simulink model "attempt_2_Full_Microthruster_Simulation"  (R2021b)
settings: Solver=ode45  StartTime=0.0  StopTime=simtime  RelTol=1e-16  AbsTol=1e-16
undefined symbols (not defined in the file): delta_t, dev_en, drag_unmodeled, dtype_g, euler_b_ECI0, euler_b_LVLH0, euler_LVLH_ECI0, g_bias, g_sath, g_satl, g_sen, g_sf_cc, geom, gr_eff_unmodeled, grav_grad_unmodeled, gyro_meas_frequ, J, JD_start, mag_field_unmodeled, mag_meas_frequ, mu, onboard_unmodeled, quat_b_ECI0, quat_b_LVLH0, quat_LVLH_ECI0, r, sigma_g, sigma_m, sigma_q, sigma_s, srp_unmodeled, sun_meas_frequ, theor_torque, ts, v, w_b_ECI0, wn, zn
libraries: aerolibnav x5, sharedTrackingLibrary x2
(part 1 of 2)
settings Model: Creator=Owner  LastModifiedBy=Owner
settings DebuggingCC: UnderSpecifiedDimensionMsg=warning

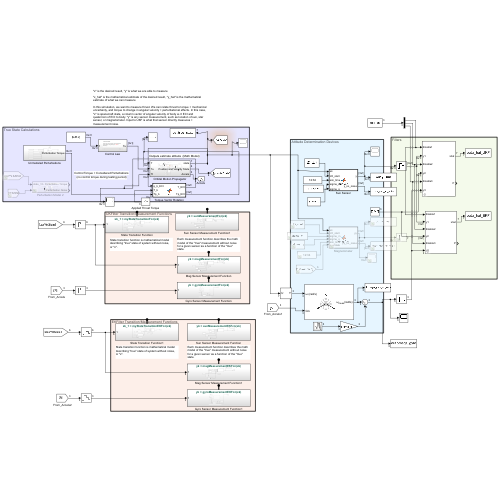
[thumbnail: Simulink's stored preview of the top-level diagram]
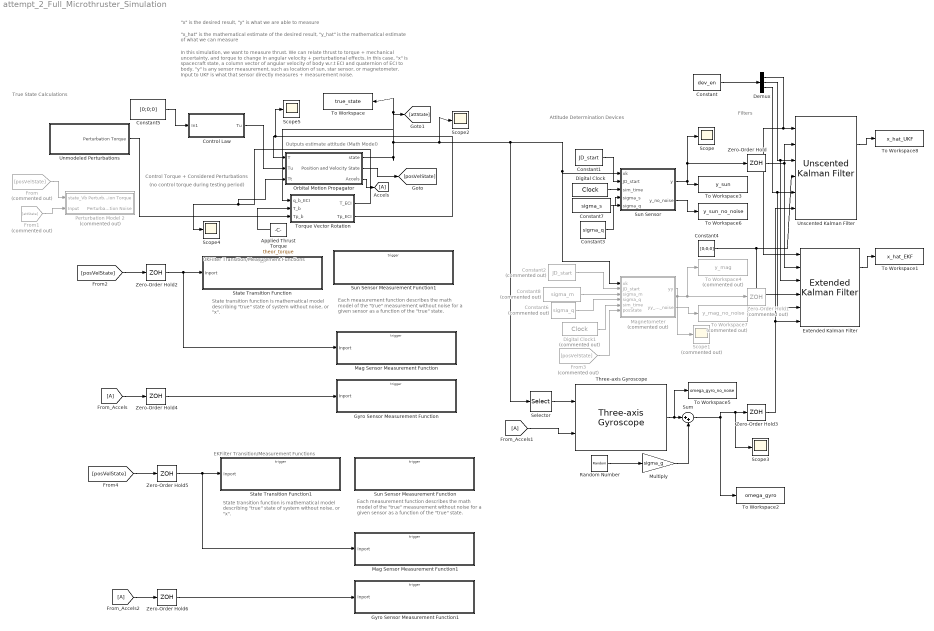
== system attempt_2_Full_Microthruster_Simulation ==
  note: Filters
  note: Attitude Determination Devices
  note: UKFilter Transition/Measurement Functions
  note: True State Calculations
  note: Each measurement function describes the math model of the "true" measurement without noise for a given sensor as a function of the "true" state.
  note: State transition function is mathematical model describing "true" state of system without noise, or "x".
  note: In this simulation, we want to measure thrust. We can relate thrust to torque + mechanical uncertainty, and torque to change in angular velocity + perturbational effects. In this case, "x" is spacecraft state, a column vector of angular velocity of body w.r.t ECI and quaternion of ECI to body. "y" is any sensor measurement, such as location of sun, star sensor, or magnetometer. Input to UKF is what that sensor directly measures + measurement noise.
  note: "x_hat" is the mathematical estimate of the desired result, "y_hat" is the mathematical estimate of what we can measure
  note: "x" is the desired result, "y" is what we are able to measure
  note: Outputs estimate attitude (Math Model)
  note: (no control torque during testing period)
  note: Control Torque + Considered Perturbations
  note: State transition function is mathematical model describing "true" state of system without noise, or "x".
  note: Each measurement function describes the math model of the "true" measurement without noise for a given sensor as a function of the "true" state.
  note: EKFilter Transition/Measurement Functions
  Applied Thrust Torque : Constant  Value=theor_torque
  Constant : Constant  Value=dev_en
  Constant1 : Constant  Value=JD_start
  Constant2 : Constant  Commented=on  Value=JD_start
  Constant3 : Constant  Value=sigma_q
  Constant4 : Constant  Value=[0;0;0]
  Constant5 : Constant  Value=[0;0;0]  VectorParams1D=off
  Constant6 : Constant  Commented=on  Value=sigma_q
  Constant7 : Constant  Value=sigma_s  VectorParams1D=off
  Constant8 : Constant  Commented=on  Value=sigma_m  VectorParams1D=off
  Control Law : Subsystem
  Demux : Demux  Outputs=3
  Digital Clock : DigitalClock  SampleTime=delta_t
  Digital Clock1 : DigitalClock  Commented=on  SampleTime=delta_t
  Extended Kalman Filter : sharedTrackingLibrary/Extended Kalman Filter  StateTransitionFcn=myStateTransitionEKFcn  HasStateTransitionJacobianFcn=off  HasAdditiveProcessNoise=Additive  ProcessNoise=Q_k  HasTimeVaryingProcessNoise=off  HasStateTransitionFcnExtraArgument=0  InitialState=x_hat0  InitialStateCovariance=P0  MeasurementFcn1=sunMeasurementEKFcn  HasMeasurementJacobianFcn1=off  HasMeasurementEnablePort1=on  HasAdditiveMeasurementNoise1=Additive  MeasurementNoise1=R_k  HasTimeVaryingMeasurementNoise1=off  HasMeasurementFcnExtraArgument1=0  MeasurementFcn2=magMeasurementEKFcn  HasMeasurementJacobianFcn2=off  HasMeasurementEnablePort2=on  HasAdditiveMeasurementNoise2=Additive  MeasurementNoise2=RR_k  HasTimeVaryingMeasurementNoise2=off  HasMeasurementFcnExtraArgument2=0  MeasurementFcn3=gyroMeasurementEKFcn  HasMeasurementJacobianFcn3=off  HasMeasurementEnablePort3=on  HasAdditiveMeasurementNoise3=Additive  MeasurementNoise3=RRR_k  HasTimeVaryingMeasurementNoise3=off  HasMeasurementFcnExtraArgument3=0  MeasurementFcn4=myMeasurementFcn  HasMeasurementJacobianFcn4=off  HasMeasurementEnablePort4=off  HasAdditiveMeasurementNoise4=Additive  MeasurementNoise4=1  HasTimeVaryingMeasurementNoise4=off  HasMeasurementFcnExtraArgument4=0  MeasurementFcn5=myMeasurementFcn  HasMeasurementJacobianFcn5=off  HasMeasurementEnablePort5=off  HasAdditiveMeasurementNoise5=Additive  MeasurementNoise5=1  HasTimeVaryingMeasurementNoise5=off  HasMeasurementFcnExtraArgument5=0  EnableMultirate=on  StateTransitionFcnSampleTime=delta_t  MeasurementFcn1SampleTime=1/sun_meas_frequ  MeasurementFcn2SampleTime=1/mag_meas_frequ  MeasurementFcn3SampleTime=1/gyro_meas_frequ  MeasurementFcn4SampleTime=1  MeasurementFcn5SampleTime=1  UseCurrentEstimator=on  OutputStateCovariance=on  DataType=double  SampleTime=delta_t  NumberOfMeasurements=3
      settings: SourceProductBaseCode=AE,PW,CT,DR,TF,ID,LP,NV,AR,RO,RR,UV,VE
  From : From  Commented=on  GotoTag=posVelState
  From1 : From  Commented=on  GotoTag=attState
  From3 : From  Commented=on  GotoTag=posVelState
  Gyro Sensor Measurement Function : Subsystem  TreatAsAtomicUnit=on
  Gyro Sensor Measurement Function1 : Subsystem  TreatAsAtomicUnit=on
  Mag Sensor Measurement Function : Subsystem  TreatAsAtomicUnit=on
  Mag Sensor Measurement Function1 : Subsystem  TreatAsAtomicUnit=on
  Magnetometer : MATLAB Function  Commented=on  TreatAsAtomicUnit=on
  Multiply : Gain  Gain=sigma_g
  Orbital Motion Propagator : Subsystem
  Perturbation Model 2 : Subsystem  Commented=on
  Random Number : RandomNumber  Seed=[0 0 0]
  Scope{,2..5} (5 alike) : Scope
  Scope1 : Scope  Commented=on
  Selector : Selector  InputPortWidth=7  IndexOptions=Index vector (dialog)  Indices=[1 2 3]  OutputSizes=1
  State Transition Function : Subsystem  TreatAsAtomicUnit=on
  State Transition Function1 : Subsystem  TreatAsAtomicUnit=on
  Sum : Sum  Inputs=|++
  Sun Sensor : MATLAB Function  TreatAsAtomicUnit=on
  Sun Sensor Measurement Function : Subsystem  TreatAsAtomicUnit=on
  Sun Sensor Measurement Function1 : Subsystem  TreatAsAtomicUnit=on
  Three-axis Gyroscope : aerolibnav/Three-axis Gyroscope  dtype_g=off  w_g=190  z_g=0.707  g_sf_cc=[1 0 0; 0 1 0; 0 0 1]  g_bias=[0 0 0]  g_sen=[0 0 0]  g_Ts=0  g_rand=off  g_seeds=[23093 23094 23095]  g_pow=[sigma_g sigma_g sigma_g]  g_sat="[-inf  -inf  -inf  inf inf inf]"
      settings: SourceProductBaseCode=AE
  To Workspace : ToWorkspace  VariableName=true_state  SaveFormat=Timeseries  SampleTime=-1
  To Workspace1 : ToWorkspace  VariableName=x_hat_EKF  SaveFormat=Timeseries  SampleTime=-1
  To Workspace2 : ToWorkspace  VariableName=omega_gyro  SaveFormat=Timeseries  SampleTime=-1
  To Workspace3 : ToWorkspace  VariableName=y_sun  SaveFormat=Timeseries  SampleTime=-1
  To Workspace4 : ToWorkspace  Commented=on  VariableName=y_mag  SaveFormat=Timeseries  SampleTime=-1
  To Workspace5 : ToWorkspace  VariableName=omega_gyro_no_noise  SaveFormat=Timeseries  SampleTime=-1
  To Workspace6 : ToWorkspace  VariableName=y_sun_no_noise  SaveFormat=Timeseries  SampleTime=-1
  To Workspace7 : ToWorkspace  Commented=on  VariableName=y_mag_no_noise  SaveFormat=Timeseries  SampleTime=-1
  To Workspace8 : ToWorkspace  VariableName=x_hat_UKF  SaveFormat=Timeseries  SampleTime=-1
  Torque Vector Rotation : MATLAB Function  TreatAsAtomicUnit=on
  Unmodeled Perturbations : Subsystem
  Unscented Kalman Filter : sharedTrackingLibrary/Unscented Kalman Filter  StateTransitionFcn=myStateTransitionFcn  HasAdditiveProcessNoise=Additive  ProcessNoise=Q_k  HasTimeVaryingProcessNoise=off  HasStateTransitionFcnExtraArgument=0  InitialState=x_hat0  InitialStateCovariance=P0  Alpha=1e-5  Beta=2  Kappa=0  MeasurementFcn1=sunMeasurementFcn  HasMeasurementEnablePort1=on  HasAdditiveMeasurementNoise1=Additive  MeasurementNoise1=R_k  HasTimeVaryingMeasurementNoise1=off  HasMeasurementFcnExtraArgument1=0  MeasurementFcn2=magMeasurementFcn  HasMeasurementEnablePort2=on  HasAdditiveMeasurementNoise2=Additive  MeasurementNoise2=RR_k  HasTimeVaryingMeasurementNoise2=off  HasMeasurementFcnExtraArgument2=0  MeasurementFcn3=gyroMeasurementFcn  HasMeasurementEnablePort3=on  HasAdditiveMeasurementNoise3=Additive  MeasurementNoise3=RRR_k  HasTimeVaryingMeasurementNoise3=off  HasMeasurementFcnExtraArgument3=0  MeasurementFcn4=myMeasurementFcn  HasMeasurementEnablePort4=off  HasAdditiveMeasurementNoise4=Nonadditive  MeasurementNoise4=1  HasTimeVaryingMeasurementNoise4=off  HasMeasurementFcnExtraArgument4=0  MeasurementFcn5=myMeasurementFcn  HasMeasurementEnablePort5=off  HasAdditiveMeasurementNoise5=Additive  MeasurementNoise5=1  HasTimeVaryingMeasurementNoise5=off  HasMeasurementFcnExtraArgument5=0  EnableMultirate=on  StateTransitionFcnSampleTime=delta_t  MeasurementFcn1SampleTime=1/sun_meas_frequ  MeasurementFcn2SampleTime=1/mag_meas_frequ  MeasurementFcn3SampleTime=1/gyro_meas_frequ  MeasurementFcn4SampleTime=1  MeasurementFcn5SampleTime=1  UseCurrentEstimator=on  OutputStateCovariance=on  DataType=double  SampleTime=delta_t  NumberOfMeasurements=3
      settings: SourceProductBaseCode=AE,PW,CT,DR,TF,ID,LP,NV,AR,RO,RR,UV,VE
  Zero-Order Hold : ZeroOrderHold  SampleTime=1/sun_meas_frequ
  Zero-Order Hold1 : ZeroOrderHold  Commented=on  SampleTime=1/mag_meas_frequ
  Zero-Order Hold{2,4..6} (4 alike) : ZeroOrderHold  SampleTime=-1
  Zero-Order Hold3 : ZeroOrderHold  SampleTime=1/gyro_meas_frequ
  wires:
  Control Law/1(Tu) -> Orbital Motion Propagator/2(Tu)
  Constant/1 -> Demux/1
  Applied Thrust Torque/1 -> Torque Vector Rotation/2(T_b)
  Torque Vector Rotation/1(T_ECI) -> Orbital Motion Propagator/3(Tt), Scope4/1
  Orbital Motion Propagator/1(state) -> Torque Vector Rotation/1(q_b_ECI), Scope2/1, Selector/1, Sun Sensor/1(xk), Magnetometer/1(xk), [attState], To Workspace/1
  Zero-Order Hold/1 -> Extended Kalman Filter/2, Unscented Kalman Filter/2
  Digital Clock/1 -> Sun Sensor/3(sim_time)
  Constant7/1 -> Sun Sensor/4(sigma_s)
  Constant1/1 -> Sun Sensor/2(JD_start)
  Constant3/1 -> Sun Sensor/5(sigma_q)
  Sun Sensor/1(y) -> To Workspace3/1, Scope/1, Zero-Order Hold/1
  Unscented Kalman Filter/1 -> To Workspace8/1
  Extended Kalman Filter/1 -> To Workspace1/1
  Constant6/1 -> Magnetometer/4(sigma_q)
  Constant8/1 -> Magnetometer/3(sigma_m)
  Magnetometer/1(yy) -> Scope1/1, Zero-Order Hold1/1, To Workspace4/1
  Orbital Motion Propagator/2(Position and Velocity State) -> [posVelState]
  From/1 -> Perturbation Model 2/1(state_Vb)
  From1/1 -> Perturbation Model 2/2(Input)
  [posVelState] -> Zero-Order Hold2/1
  Digital Clock1/1 -> Magnetometer/5(sim_time)
  From3/1 -> Magnetometer/6(posState)
  Zero-Order Hold2/1 -> Mag Sensor Measurement Function/1(Inport), State Transition Function/1(Inport)
  Constant5/1 -> Control Law/1(In1)
  Selector/1 -> Three-axis Gyroscope/1
  Zero-Order Hold3/1 -> Unscented Kalman Filter/6, Extended Kalman Filter/6
  Orbital Motion Propagator/3(Accels) -> [A]
  [A] -> Zero-Order Hold4/1
  Zero-Order Hold4/1 -> Gyro Sensor Measurement Function/1(Inport)
  [A] -> Three-axis Gyroscope/2
  Zero-Order Hold6/1 -> Gyro Sensor Measurement Function1/1(Inport)
  Zero-Order Hold5/1 -> Mag Sensor Measurement Function1/1(Inport), State Transition Function1/1(Inport)
  [A] -> Zero-Order Hold6/1
  [posVelState] -> Zero-Order Hold5/1
  Random Number/1 -> Multiply/1
  Multiply/1 -> Sum/2
  Three-axis Gyroscope/1 -> To Workspace5/1, Sum/1
  Sum/1 -> Scope3/1, Zero-Order Hold3/1, To Workspace2/1
  Constant2/1 -> Magnetometer/2(JD_start)
  Sun Sensor/2(y_no_noise) -> To Workspace6/1
  Magnetometer/2(yy_no_noise) -> To Workspace7/1
  Demux/3 -> Unscented Kalman Filter/5, Extended Kalman Filter/5
  Demux/2 -> Extended Kalman Filter/3, Unscented Kalman Filter/3
  Demux/1 -> Unscented Kalman Filter/1, Extended Kalman Filter/1
  Unmodeled Perturbations/1(Perturbation Torque) -> Torque Vector Rotation/3(Tp_b)
  Torque Vector Rotation/2(Tp_ECI) -> Scope5/1, Orbital Motion Propagator/1(T)
  Constant4/1 -> Unscented Kalman Filter/4, Extended Kalman Filter/4

== system attempt_2_Full_Microthruster_Simulation/Control Law ==
  note: PLACEHOLDER:
      |
      | Likely only control device on board will be impermanent magnetorquer; TBM if necessary
  In1 : Inport
  Tu : Outport
  wires:
  In1/1 -> Tu/1

== system attempt_2_Full_Microthruster_Simulation/Gyro Sensor Measurement Function ==
  note: Identical to "three-axis gyroscope" block, except modified to inherit sample time
  Inport : Inport
  gyroMeasurementFcn : TriggerPort  TriggerType=function-call  IsSimulinkFunction=on  FunctionName=gyroMeasurementFcn  FunctionVisibility=scoped  VariantControl=(inherit)
  Scope : Scope
  Selector : Selector  InputPortWidth=7  IndexOptions=Index vector (dialog)  Indices=[1 2 3]  OutputSizes=1
  Subsystem : Subsystem
  Three-axis Gyroscope : aerolibnav/Three-axis Gyroscope  Commented=on  dtype_g=on  w_g=190  z_g=0.707  g_sf_cc=[1 0 0; 0 1 0; 0 0 1]  g_bias=[0 0 0]  g_sen=[0 0 0]  g_Ts=1/gyro_meas_frequ  g_rand=off  g_seeds=[23093 23094 23095]  g_pow=[0.0001 0.0001 0.0001]  g_sat="[-inf  -inf  -inf  inf inf inf]"
      settings: SourceProductBaseCode=AE
  To Workspace : ToWorkspace  VariableName=y_UKF_gyro  SaveFormat=Timeseries  SampleTime=-1
  xk : ArgIn  DisableCoverage=on  PortDimensions=[7 1]  ArgumentName=xk
  yk : ArgOut  DisableCoverage=on  PortDimensions=[3 1]  ArgumentName=yk
  wires:
  Selector/1 -> Subsystem/1(p q r)
  xk/1 -> Selector/1
  Inport/1 -> Subsystem/2(G's)
  Subsystem/1((p q r)_meas) -> Scope/1, To Workspace/1, yk/1

== system attempt_2_Full_Microthruster_Simulation/Gyro Sensor Measurement Function1 ==
  note: Identical to "three-axis gyroscope" block, except modified to inherit sample time
  Inport : Inport
  gyroMeasurementEKFcn : TriggerPort  TriggerType=function-call  IsSimulinkFunction=on  FunctionName=gyroMeasurementEKFcn  FunctionVisibility=scoped  VariantControl=(inherit)
  Scope : Scope
  Selector : Selector  InputPortWidth=7  IndexOptions=Index vector (dialog)  Indices=[1 2 3]  OutputSizes=1
  Subsystem : Subsystem
  Three-axis Gyroscope : aerolibnav/Three-axis Gyroscope  Commented=on  dtype_g=on  w_g=190  z_g=0.707  g_sf_cc=[1 0 0; 0 1 0; 0 0 1]  g_bias=[0 0 0]  g_sen=[0 0 0]  g_Ts=1/gyro_meas_frequ  g_rand=off  g_seeds=[23093 23094 23095]  g_pow=[0.0001 0.0001 0.0001]  g_sat="[-inf  -inf  -inf  inf inf inf]"
      settings: SourceProductBaseCode=AE
  To Workspace : ToWorkspace  VariableName=y_EKF_gyro  SaveFormat=Timeseries  SampleTime=-1
  xk : ArgIn  DisableCoverage=on  PortDimensions=[7 1]  ArgumentName=xk
  yk : ArgOut  DisableCoverage=on  PortDimensions=[3 1]  ArgumentName=yk
  wires:
  Selector/1 -> Subsystem/1(p q r)
  xk/1 -> Selector/1
  Inport/1 -> Subsystem/2(G's)
  Subsystem/1((p q r)_meas) -> Scope/1, To Workspace/1, yk/1

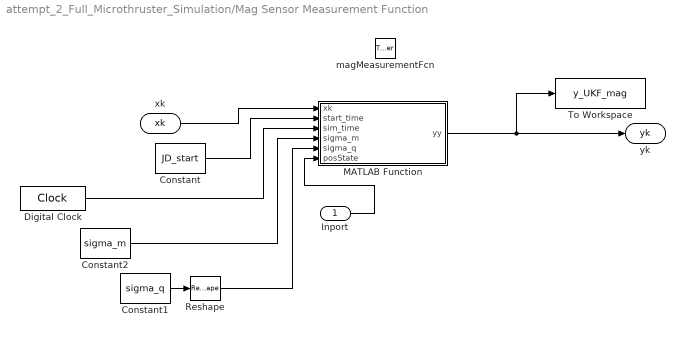
== system attempt_2_Full_Microthruster_Simulation/Mag Sensor Measurement Function ==
  Inport : Inport
  magMeasurementFcn : TriggerPort  TriggerType=function-call  IsSimulinkFunction=on  FunctionName=magMeasurementFcn  FunctionVisibility=scoped  VariantControl=(inherit)
  Constant : Constant  Value=JD_start
  Constant1 : Constant  Value=sigma_q  VectorParams1D=off  SampleTime=-1
  Constant2 : Constant  Value=sigma_m  VectorParams1D=off  SampleTime=-1
  Digital Clock : DigitalClock  SampleTime=-1
  MATLAB Function : MATLAB Function  TreatAsAtomicUnit=on
  Reshape : Reshape
  To Workspace : ToWorkspace  VariableName=y_UKF_mag  SaveFormat=Timeseries  SampleTime=-1
  xk : ArgIn  DisableCoverage=on  PortDimensions=[7 1]  ArgumentName=xk
  yk : ArgOut  DisableCoverage=on  PortDimensions=[3 1]  ArgumentName=yk
  wires:
  xk/1 -> MATLAB Function/1(xk)
  MATLAB Function/1(yy) -> To Workspace/1, yk/1
  Constant/1 -> MATLAB Function/2(start_time)
  Digital Clock/1 -> MATLAB Function/3(sim_time)
  Constant2/1 -> MATLAB Function/4(sigma_m)
  Constant1/1 -> Reshape/1
  Reshape/1 -> MATLAB Function/5(sigma_q)
  Inport/1 -> MATLAB Function/6(posState)

== system attempt_2_Full_Microthruster_Simulation/Mag Sensor Measurement Function1 ==
  Inport : Inport
  magMeasurementEKFcn : TriggerPort  TriggerType=function-call  IsSimulinkFunction=on  FunctionName=magMeasurementEKFcn  FunctionVisibility=scoped  VariantControl=(inherit)
  Constant : Constant  Value=JD_start
  Constant1 : Constant  Value=sigma_q  VectorParams1D=off  SampleTime=-1
  Constant2 : Constant  Value=sigma_m  VectorParams1D=off  SampleTime=-1
  Digital Clock : DigitalClock  SampleTime=-1
  MATLAB Function : MATLAB Function  TreatAsAtomicUnit=on
  Reshape : Reshape
  To Workspace : ToWorkspace  VariableName=y_EKF_mag  SaveFormat=Timeseries  SampleTime=-1
  xk : ArgIn  DisableCoverage=on  PortDimensions=[7 1]  ArgumentName=xk
  yk : ArgOut  DisableCoverage=on  PortDimensions=[3 1]  ArgumentName=yk
  wires:
  xk/1 -> MATLAB Function/1(xk)
  MATLAB Function/1(yy) -> To Workspace/1, yk/1
  Constant/1 -> MATLAB Function/2(JD_start)
  Digital Clock/1 -> MATLAB Function/3(sim_time)
  Constant2/1 -> MATLAB Function/4(sigma_m)
  Constant1/1 -> Reshape/1
  Reshape/1 -> MATLAB Function/5(sigma_q)
  Inport/1 -> MATLAB Function/6(posState)

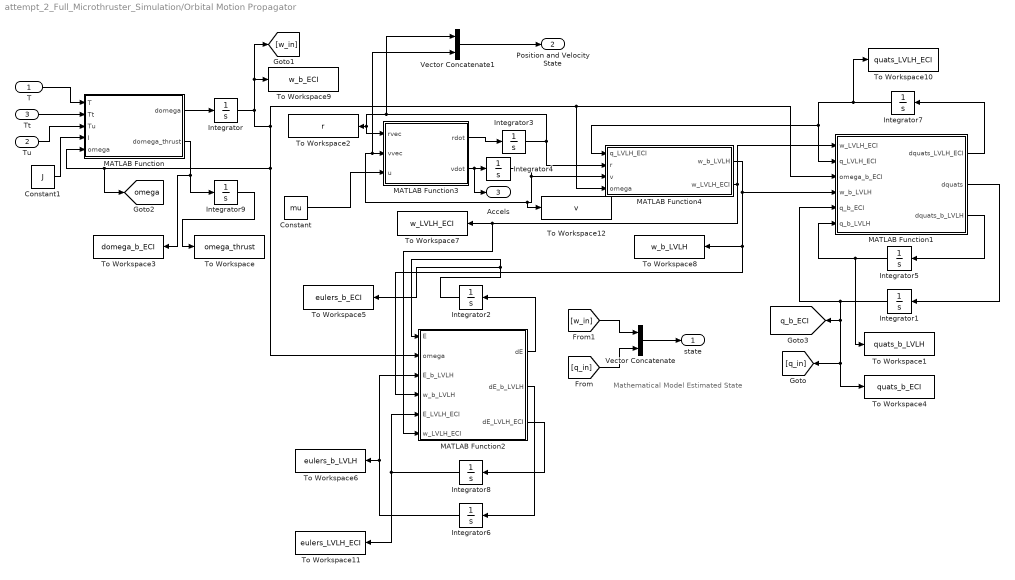
== system attempt_2_Full_Microthruster_Simulation/Orbital Motion Propagator ==
  note: Mathematical Model Estimated State
  T : Inport
  Tu : Inport  Port=2
  Tt : Inport  Port=3
  Constant : Constant  Value=mu
  Constant1 : Constant  Value=J
  Integrator : Integrator  InitialCondition=w_b_ECI0
  Integrator1 : Integrator  InitialCondition=quat_b_ECI0
  Integrator2 : Integrator  InitialCondition=euler_b_ECI0
  Integrator3 : Integrator  InitialCondition=r
  Integrator4 : Integrator  InitialCondition=v
  Integrator5 : Integrator  InitialCondition=quat_b_LVLH0
  Integrator6 : Integrator  InitialCondition=euler_b_LVLH0
  Integrator7 : Integrator  InitialCondition=quat_LVLH_ECI0
  Integrator8 : Integrator  InitialCondition=euler_LVLH_ECI0
  Integrator9 : Integrator  InitialCondition=w_b_ECI0
  MATLAB Function : MATLAB Function  TreatAsAtomicUnit=on
  MATLAB Function1 : MATLAB Function  TreatAsAtomicUnit=on
  MATLAB Function2 : MATLAB Function  TreatAsAtomicUnit=on
  MATLAB Function3 : MATLAB Function  TreatAsAtomicUnit=on
  MATLAB Function4 : MATLAB Function  TreatAsAtomicUnit=on
  To Workspace : ToWorkspace  VariableName=omega_thrust  SaveFormat=Timeseries  SampleTime=-1
  To Workspace1 : ToWorkspace  VariableName=quats_b_LVLH  SaveFormat=Timeseries  SampleTime=-1
  To Workspace10 : ToWorkspace  VariableName=quats_LVLH_ECI  SaveFormat=Timeseries  SampleTime=-1
  To Workspace11 : ToWorkspace  VariableName=eulers_LVLH_ECI  SaveFormat=Timeseries  SampleTime=-1
  To Workspace12 : ToWorkspace  VariableName=v  SaveFormat=Timeseries  SampleTime=-1
  To Workspace2 : ToWorkspace  VariableName=r  SaveFormat=Timeseries  SampleTime=-1
  To Workspace3 : ToWorkspace  VariableName=domega_b_ECI  SaveFormat=Timeseries  SampleTime=-1
  To Workspace4 : ToWorkspace  VariableName=quats_b_ECI  SaveFormat=Timeseries  SampleTime=-1
  To Workspace5 : ToWorkspace  VariableName=eulers_b_ECI  SaveFormat=Timeseries  SampleTime=-1
  To Workspace6 : ToWorkspace  VariableName=eulers_b_LVLH  SaveFormat=Timeseries  SampleTime=-1
  To Workspace7 : ToWorkspace  VariableName=w_LVLH_ECI  SaveFormat=Timeseries  SampleTime=-1
  To Workspace8 : ToWorkspace  VariableName=w_b_LVLH  SaveFormat=Timeseries  SampleTime=-1
  To Workspace9 : ToWorkspace  VariableName=w_b_ECI  SaveFormat=Timeseries  SampleTime=-1
  Vector Concatenate : Concatenate  Mode=Multidimensional array
  Vector Concatenate1 : Concatenate
  state : Outport
  Position and Velocity State : Outport  Port=2
  Accels : Outport  Port=3
  tag scope: omega=global, q_b_ECI=global
  wires:
  MATLAB Function1/2(dquats) -> Integrator1/1
  MATLAB Function2/1(dE) -> Integrator2/1
  Integrator6/1 -> To Workspace6/1, MATLAB Function2/3(E_b_LVLH)
  MATLAB Function3/2(vdot) -> Accels/1, Integrator4/1
  Integrator5/1 -> MATLAB Function1/6(q_b_LVLH), To Workspace1/1
  MATLAB Function1/3(dquats_b_LVLH) -> Integrator5/1
  Integrator7/1 -> To Workspace10/1, MATLAB Function4/1(q_LVLH_ECI), MATLAB Function1/2(q_LVLH_ECI)
  Integrator/1 -> [omega], MATLAB Function/5(omega), MATLAB Function2/2(omega), MATLAB Function4/4(omega), MATLAB Function1/3(omega_b_ECI), [w_in], To Workspace9/1
  MATLAB Function3/1(rdot) -> Integrator3/1
  T/1 -> MATLAB Function/1(T)
  MATLAB Function4/2(w_LVLH_ECI) -> MATLAB Function1/1(w_LVLH_ECI), MATLAB Function2/6(w_LVLH_ECI), To Workspace7/1
  MATLAB Function2/2(dE_b_LVLH) -> Integrator6/1
  Integrator1/1 -> MATLAB Function1/5(q_b_ECI), To Workspace4/1, [q_in], [q_b_ECI]
  MATLAB Function/1(domega) -> Integrator/1
  MATLAB Function4/1(w_b_LVLH) -> MATLAB Function2/4(w_b_LVLH), To Workspace8/1, MATLAB Function1/4(w_b_LVLH)
  Integrator8/1 -> To Workspace11/1, MATLAB Function2/5(E_LVLH_ECI)
  Integrator2/1 -> To Workspace5/1, MATLAB Function2/1(E)
  MATLAB Function1/1(dquats_LVLH_ECI) -> Integrator7/1
  Constant1/1 -> MATLAB Function/4(I)
  MATLAB Function2/3(dE_LVLH_ECI) -> Integrator8/1
  Vector Concatenate/1 -> state/1
  [q_in] -> Vector Concatenate/2
  [w_in] -> Vector Concatenate/1
  Integrator3/1 -> Vector Concatenate1/1, To Workspace2/1, MATLAB Function3/1(rvec), MATLAB Function4/2(r)
  Vector Concatenate1/1 -> Position and Velocity State/1
  Integrator4/1 -> MATLAB Function4/3(v), To Workspace12/1, Vector Concatenate1/2, MATLAB Function3/2(vvec)
  Tt/1 -> MATLAB Function/2(Tt)
  Tu/1 -> MATLAB Function/3(Tu)
  MATLAB Function/2(domega_thrust) -> Integrator9/1, To Workspace3/1
  Integrator9/1 -> To Workspace/1
  Constant/1 -> MATLAB Function3/3(u)

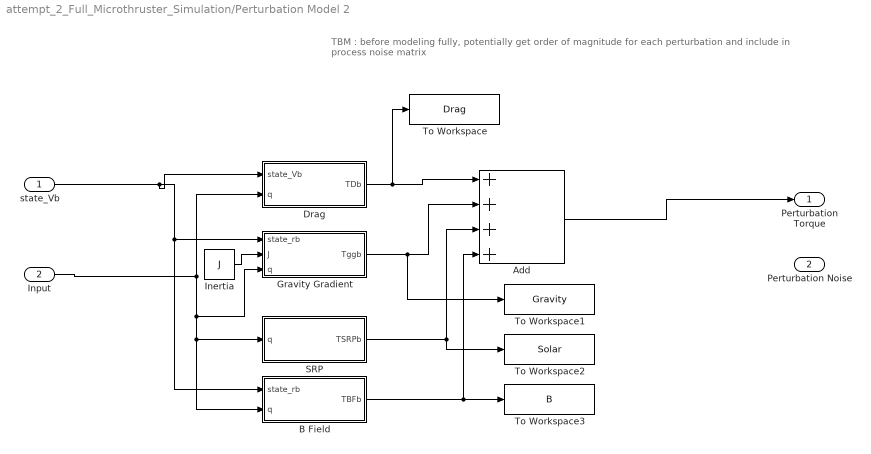
== system attempt_2_Full_Microthruster_Simulation/Perturbation Model 2 ==
  note: TBM : before modeling fully, potentially get order of magnitude for each perturbation and include in process noise matrix
  state_Vb : Inport
  Input : Inport  Port=2
  Add : Sum  Inputs=++++
  B Field : Subsystem
  Drag : Subsystem
  Gravity Gradient : Subsystem
  Inertia : Constant  Value=J
  SRP : Subsystem
  To Workspace : ToWorkspace  VariableName=Drag  SaveFormat=Timeseries  SampleTime=-1
  To Workspace1 : ToWorkspace  VariableName=Gravity  SaveFormat=Timeseries  SampleTime=-1
  To Workspace2 : ToWorkspace  VariableName=Solar  SaveFormat=Timeseries  SampleTime=-1
  To Workspace3 : ToWorkspace  VariableName=B  SaveFormat=Timeseries  SampleTime=-1
  Perturbation Torque : Outport
  Perturbation Noise : Outport  Port=2
  wires:
  B Field/1(TBFb) -> To Workspace3/1, Add/4
  Drag/1(TDb) -> To Workspace/1, Add/1
  Input/1 -> B Field/2(q), SRP/1(q), Gravity Gradient/3(q), Drag/2(q)
  Inertia/1 -> Gravity Gradient/2(J)
  Gravity Gradient/1(Tggb) -> To Workspace1/1, Add/2
  state_Vb/1 -> B Field/1(state_rb), Gravity Gradient/1(state_rb), Drag/1(state_Vb)
  SRP/1(TSRPb) -> To Workspace2/1, Add/3
  Add/1 -> Perturbation Torque/1

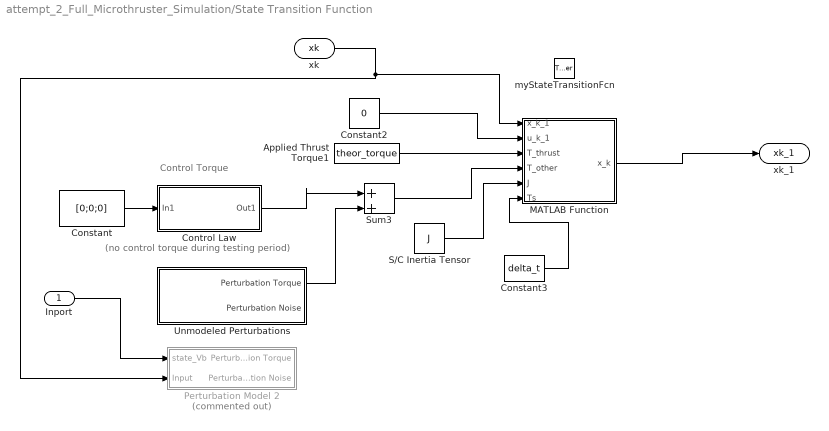
== system attempt_2_Full_Microthruster_Simulation/State Transition Function ==
  note: Control Torque
  note: (no control torque during testing period)
  Inport : Inport
  myStateTransitionFcn : TriggerPort  TriggerType=function-call  IsSimulinkFunction=on  FunctionName=myStateTransitionFcn  FunctionVisibility=scoped  VariantControl=(inherit)
  Applied Thrust Torque1 : Constant  Value=theor_torque
  Constant : Constant  Value=[0;0;0]  VectorParams1D=off
  Constant2 : Constant  Value=0
  Constant3 : Constant  Value=delta_t
  Control Law : Subsystem
  MATLAB Function : MATLAB Function  TreatAsAtomicUnit=on
  Perturbation Model 2 : Subsystem  Commented=on
  S/C Inertia Tensor : Constant  Value=J
  Sum3 : Sum  Inputs=+|+
  Unmodeled Perturbations : Subsystem
  xk : ArgIn  DisableCoverage=on  PortDimensions=[7 1]  ArgumentName=xk
  xk_1 : ArgOut  DisableCoverage=on  PortDimensions=[7 1]  ArgumentName=xk_1
  wires:
  Control Law/1(Out1) -> Sum3/1
  Unmodeled Perturbations/1(Perturbation Torque) -> Sum3/2
  MATLAB Function/1(x_k) -> xk_1/1
  Applied Thrust Torque1/1 -> MATLAB Function/3(T_thrust)
  Sum3/1 -> MATLAB Function/4(T_other)
  Constant2/1 -> MATLAB Function/2(u_k_1)
  Constant/1 -> Control Law/1(In1)
  S/C Inertia Tensor/1 -> MATLAB Function/5(J)
  Constant3/1 -> MATLAB Function/6(Ts)
  xk/1 -> Perturbation Model 2/2(Input), MATLAB Function/1(x_k_1)
  Inport/1 -> Perturbation Model 2/1(state_Vb)

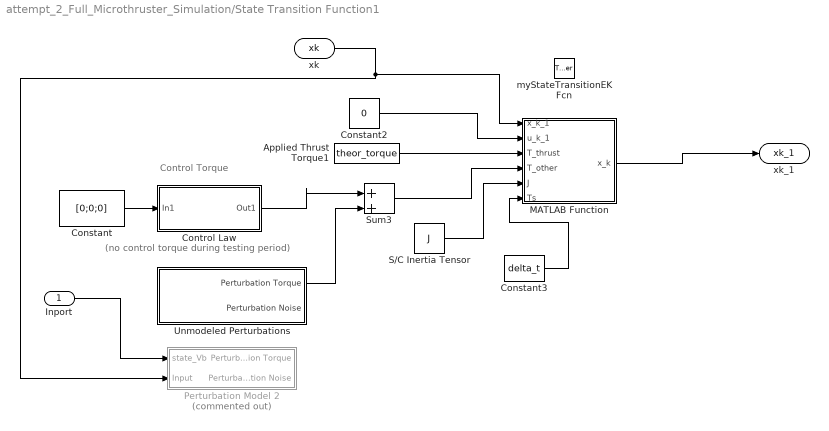
== system attempt_2_Full_Microthruster_Simulation/State Transition Function1 ==
  note: Control Torque
  note: (no control torque during testing period)
  Inport : Inport
  myStateTransitionEKFcn : TriggerPort  TriggerType=function-call  IsSimulinkFunction=on  FunctionName=myStateTransitionEKFcn  FunctionVisibility=scoped  VariantControl=(inherit)
  Applied Thrust Torque1 : Constant  Value=theor_torque
  Constant : Constant  Value=[0;0;0]  VectorParams1D=off
  Constant2 : Constant  Value=0
  Constant3 : Constant  Value=delta_t
  Control Law : Subsystem
  MATLAB Function : MATLAB Function  TreatAsAtomicUnit=on
  Perturbation Model 2 : Subsystem  Commented=on
  S/C Inertia Tensor : Constant  Value=J
  Sum3 : Sum  Inputs=+|+
  Unmodeled Perturbations : Subsystem
  xk : ArgIn  DisableCoverage=on  PortDimensions=[7 1]  ArgumentName=xk
  xk_1 : ArgOut  DisableCoverage=on  PortDimensions=[7 1]  ArgumentName=xk_1
  wires:
  Control Law/1(Out1) -> Sum3/1
  Unmodeled Perturbations/1(Perturbation Torque) -> Sum3/2
  MATLAB Function/1(x_k) -> xk_1/1
  Applied Thrust Torque1/1 -> MATLAB Function/3(T_thrust)
  Sum3/1 -> MATLAB Function/4(T_other)
  Constant2/1 -> MATLAB Function/2(u_k_1)
  Constant/1 -> Control Law/1(In1)
  S/C Inertia Tensor/1 -> MATLAB Function/5(J)
  Constant3/1 -> MATLAB Function/6(Ts)
  xk/1 -> Perturbation Model 2/2(Input), MATLAB Function/1(x_k_1)
  Inport/1 -> Perturbation Model 2/1(state_Vb)

== system attempt_2_Full_Microthruster_Simulation/Sun Sensor Measurement Function ==
  sunMeasurementEKFcn : TriggerPort  TriggerType=function-call  IsSimulinkFunction=on  FunctionName=sunMeasurementEKFcn  FunctionVisibility=scoped  VariantControl=(inherit)
  Constant : Constant  Value=JD_start
  Constant1 : Constant  Value=sigma_q  VectorParams1D=off  SampleTime=-1
  Constant2 : Constant  Value=sigma_s  VectorParams1D=off  SampleTime=-1
  Digital Clock : DigitalClock  SampleTime=-1
  MATLAB Function : MATLAB Function  TreatAsAtomicUnit=on
  Reshape : Reshape
  To Workspace : ToWorkspace  VariableName=y_EKF_sun  SaveFormat=Timeseries  SampleTime=-1
  xk : ArgIn  DisableCoverage=on  PortDimensions=[7 1]  ArgumentName=xk
  yk : ArgOut  DisableCoverage=on  PortDimensions=[3 1]  ArgumentName=yk
  wires:
  xk/1 -> MATLAB Function/1(xk)
  MATLAB Function/1(y) -> To Workspace/1, yk/1
  Constant/1 -> MATLAB Function/2(start_time)
  Digital Clock/1 -> MATLAB Function/3(sim_time)
  Constant2/1 -> MATLAB Function/4(sigma_s)
  Constant1/1 -> Reshape/1
  Reshape/1 -> MATLAB Function/5(sigma_q)

== system attempt_2_Full_Microthruster_Simulation/Sun Sensor Measurement Function1 ==
  sunMeasurementFcn : TriggerPort  TriggerType=function-call  IsSimulinkFunction=on  FunctionName=sunMeasurementFcn  FunctionVisibility=scoped  VariantControl=(inherit)
  Constant : Constant  Value=JD_start
  Constant1 : Constant  Value=sigma_q  VectorParams1D=off  SampleTime=-1
  Constant2 : Constant  Value=sigma_s  VectorParams1D=off  SampleTime=-1
  Digital Clock : DigitalClock  SampleTime=-1
  MATLAB Function : MATLAB Function  TreatAsAtomicUnit=on
  Reshape : Reshape
  Scope : Scope
  To Workspace : ToWorkspace  VariableName=y_UKF_sun  SaveFormat=Timeseries  SampleTime=-1
  xk : ArgIn  DisableCoverage=on  PortDimensions=[7 1]  ArgumentName=xk
  yk : ArgOut  DisableCoverage=on  PortDimensions=[3 1]  ArgumentName=yk
  wires:
  xk/1 -> MATLAB Function/1(xk)
  MATLAB Function/1(y) -> To Workspace/1, Scope/1, yk/1
  Constant/1 -> MATLAB Function/2(start_time)
  Digital Clock/1 -> MATLAB Function/3(sim_time)
  Constant2/1 -> MATLAB Function/4(sigma_s)
  Constant1/1 -> Reshape/1
  Reshape/1 -> MATLAB Function/5(sigma_q)

== system attempt_2_Full_Microthruster_Simulation/Unmodeled Perturbations ==
  Add : Sum  Inputs=++++++
  Constant : Constant  Value=drag_unmodeled  VectorParams1D=off
  Constant1 : Constant  Value=grav_grad_unmodeled  VectorParams1D=off
  Constant2 : Constant  Value=mag_field_unmodeled  VectorParams1D=off
  Constant3 : Constant  Value=srp_unmodeled  VectorParams1D=off
  Constant4 : Constant  Value=gr_eff_unmodeled  VectorParams1D=off
  Constant5 : Constant  Value=onboard_unmodeled  VectorParams1D=off
  Scope : Scope
  Perturbation Torque : Outport
  wires:
  Constant/1 -> Add/1
  Constant1/1 -> Add/2
  Constant2/1 -> Add/3
  Constant3/1 -> Add/4
  Constant4/1 -> Add/5
  Constant5/1 -> Add/6
  Add/1 -> Scope/1, Perturbation Torque/1

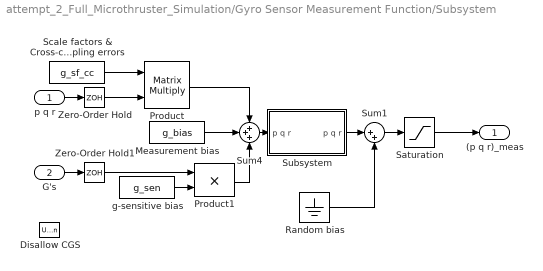
== system attempt_2_Full_Microthruster_Simulation/Gyro Sensor Measurement Function/Subsystem ==
  p q r : Inport  Unit=rad/s  PortDimensions=3
  G's : Inport  Port=2  Unit=gn  PortDimensions=3
  Disallow CGS : UnitConfiguration  UnitSystemsStr=English,SI,SI (extended)  AllowAllUnitSystems=off
  Measurement bias : Constant  Value=g_bias
  Product : Product  Multiplication=Matrix(*)  SaturateOnIntegerOverflow=on  OutDataTypeStr=Inherit: Same as first input
  Product1 : Product  SaturateOnIntegerOverflow=on  OutDataTypeStr=Inherit: Same as first input
  Random bias : Ground
  Saturation : Saturate  UpperLimit=g_sath  LowerLimit=g_satl
  "Scale factors & Cross-coupling errors " : Constant  Value=g_sf_cc
  Subsystem : Subsystem
  Sum1 : Sum  Inputs=|++  SaturateOnIntegerOverflow=on
  Sum4 : Sum  Inputs=+++  SaturateOnIntegerOverflow=on
  Zero-Order Hold : ZeroOrderHold  SampleTime=-1
  Zero-Order Hold1 : ZeroOrderHold  SampleTime=-1
  g-sensitive bias : Constant  Value=g_sen
  (p q r)_meas : Outport  Unit=rad/s  PortDimensions=3  VectorParamsAs1DForOutWhenUnconnected=off
  wires:
  Zero-Order Hold1/1 -> Product1/1
  Product1/1 -> Sum4/3
  p q r/1 -> Zero-Order Hold/1
  Zero-Order Hold/1 -> Product/2
  Sum1/1 -> Saturation/1
  g-sensitive bias/1 -> Product1/2
  "Scale factors & Cross-coupling errors "/1 -> Product/1
  G's/1 -> Zero-Order Hold1/1
  Random bias/1 -> Sum1/2
  Product/1 -> Sum4/1
  Measurement bias/1 -> Sum4/2
  Saturation/1 -> (p q r)_meas/1
  Sum4/1 -> Subsystem/1(p q r)
  Subsystem/1("p q r ") -> Sum1/1

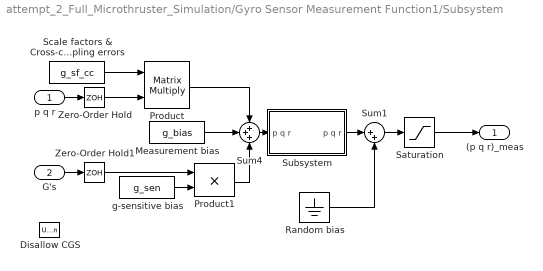
== system attempt_2_Full_Microthruster_Simulation/Gyro Sensor Measurement Function1/Subsystem ==
  p q r : Inport  Unit=rad/s  PortDimensions=3
  G's : Inport  Port=2  Unit=gn  PortDimensions=3
  Disallow CGS : UnitConfiguration  UnitSystemsStr=English,SI,SI (extended)  AllowAllUnitSystems=off
  Measurement bias : Constant  Value=g_bias
  Product : Product  Multiplication=Matrix(*)  SaturateOnIntegerOverflow=on  OutDataTypeStr=Inherit: Same as first input
  Product1 : Product  SaturateOnIntegerOverflow=on  OutDataTypeStr=Inherit: Same as first input
  Random bias : Ground
  Saturation : Saturate  UpperLimit=g_sath  LowerLimit=g_satl
  "Scale factors & Cross-coupling errors " : Constant  Value=g_sf_cc
  Subsystem : Subsystem
  Sum1 : Sum  Inputs=|++  SaturateOnIntegerOverflow=on
  Sum4 : Sum  Inputs=+++  SaturateOnIntegerOverflow=on
  Zero-Order Hold : ZeroOrderHold  SampleTime=-1
  Zero-Order Hold1 : ZeroOrderHold  SampleTime=-1
  g-sensitive bias : Constant  Value=g_sen
  (p q r)_meas : Outport  Unit=rad/s  PortDimensions=3  VectorParamsAs1DForOutWhenUnconnected=off
  wires:
  Zero-Order Hold1/1 -> Product1/1
  Product1/1 -> Sum4/3
  p q r/1 -> Zero-Order Hold/1
  Zero-Order Hold/1 -> Product/2
  Sum1/1 -> Saturation/1
  g-sensitive bias/1 -> Product1/2
  "Scale factors & Cross-coupling errors "/1 -> Product/1
  G's/1 -> Zero-Order Hold1/1
  Random bias/1 -> Sum1/2
  Product/1 -> Sum4/1
  Measurement bias/1 -> Sum4/2
  Saturation/1 -> (p q r)_meas/1
  Sum4/1 -> Subsystem/1(p q r)
  Subsystem/1("p q r ") -> Sum1/1

== system attempt_2_Full_Microthruster_Simulation/Perturbation Model 2/B Field ==
  state_rb : Inport
  q : Inport  Port=2
  Clock : Clock
  MATLAB Function : MATLAB Function  TreatAsAtomicUnit=on
  Tb : Scope
  TBFb : Outport
  wires:
  state_rb/1 -> MATLAB Function/1(state_rb)
  q/1 -> MATLAB Function/2(attState)
  MATLAB Function/1(Tmb) -> Tb/1, TBFb/1
  Clock/1 -> MATLAB Function/3(t)

== system attempt_2_Full_Microthruster_Simulation/Perturbation Model 2/Drag ==
  state_Vb : Inport
  q : Inport  Port=2
  Constant : Constant  Value=geom
  MATLAB Function : MATLAB Function  TreatAsAtomicUnit=on
  Tdrag : Scope
  TDb : Outport
  wires:
  state_Vb/1 -> MATLAB Function/1(state)
  q/1 -> MATLAB Function/2(attState)
  MATLAB Function/1(Td) -> Tdrag/1, TDb/1
  Constant/1 -> MATLAB Function/3(geom)

== system attempt_2_Full_Microthruster_Simulation/Perturbation Model 2/Gravity Gradient ==
  state_rb : Inport
  J : Inport  Port=2
  q : Inport  Port=3
  MATLAB Function : MATLAB Function  TreatAsAtomicUnit=on
  Tgg : Scope
  Tggb : Outport
  wires:
  state_rb/1 -> MATLAB Function/2(state_rb)
  J/1 -> MATLAB Function/1(J)
  MATLAB Function/1(Tgg) -> Tgg/1, Tggb/1
  q/1 -> MATLAB Function/3(attState)

== system attempt_2_Full_Microthruster_Simulation/Perturbation Model 2/SRP ==
  q : Inport
  Constant : Constant  Value=geom
  MATLAB Function : MATLAB Function  TreatAsAtomicUnit=on
  Tsrp : Scope
  TSRPb : Outport
  wires:
  MATLAB Function/1(Tsrp) -> Tsrp/1, TSRPb/1
  q/1 -> MATLAB Function/1(attState)
  Constant/1 -> MATLAB Function/2(geom)

== system attempt_2_Full_Microthruster_Simulation/State Transition Function/Control Law ==
  note: PLACEHOLDER:
      |
      | Likely only control device on board will be impermanent magnetorquer; TBM if necessary, otherwise leave as zero vector
  In1 : Inport
  Out1 : Outport
  wires:
  In1/1 -> Out1/1

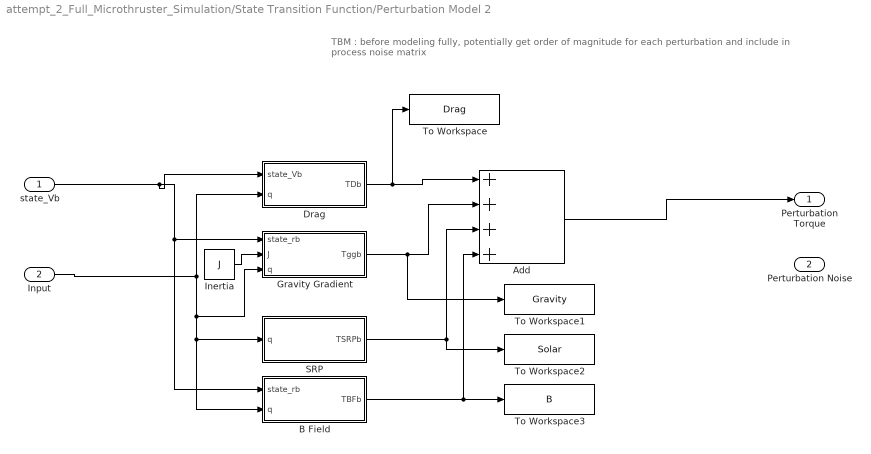
== system attempt_2_Full_Microthruster_Simulation/State Transition Function/Perturbation Model 2 ==
  note: TBM : before modeling fully, potentially get order of magnitude for each perturbation and include in process noise matrix
  state_Vb : Inport
  Input : Inport  Port=2
  Add : Sum  Inputs=++++
  B Field : Subsystem
  Drag : Subsystem
  Gravity Gradient : Subsystem
  Inertia : Constant  Value=J
  SRP : Subsystem
  To Workspace : ToWorkspace  VariableName=Drag  SaveFormat=Timeseries  SampleTime=-1
  To Workspace1 : ToWorkspace  VariableName=Gravity  SaveFormat=Timeseries  SampleTime=-1
  To Workspace2 : ToWorkspace  VariableName=Solar  SaveFormat=Timeseries  SampleTime=-1
  To Workspace3 : ToWorkspace  VariableName=B  SaveFormat=Timeseries  SampleTime=-1
  Perturbation Torque : Outport
  Perturbation Noise : Outport  Port=2
  wires:
  B Field/1(TBFb) -> To Workspace3/1, Add/4
  Drag/1(TDb) -> To Workspace/1, Add/1
  Input/1 -> B Field/2(q), SRP/1(q), Gravity Gradient/3(q), Drag/2(q)
  Inertia/1 -> Gravity Gradient/2(J)
  Gravity Gradient/1(Tggb) -> To Workspace1/1, Add/2
  state_Vb/1 -> B Field/1(state_rb), Gravity Gradient/1(state_rb), Drag/1(state_Vb)
  SRP/1(TSRPb) -> To Workspace2/1, Add/3
  Add/1 -> Perturbation Torque/1

== system attempt_2_Full_Microthruster_Simulation/State Transition Function/Unmodeled Perturbations ==
  Add : Sum  Inputs=++++++
  Constant : Constant  Value=drag_unmodeled  VectorParams1D=off
  Constant1 : Constant  Value=grav_grad_unmodeled  VectorParams1D=off
  Constant2 : Constant  Value=mag_field_unmodeled  VectorParams1D=off
  Constant3 : Constant  Value=srp_unmodeled  VectorParams1D=off
  Constant4 : Constant  Value=gr_eff_unmodeled  VectorParams1D=off
  Constant5 : Constant  Value=onboard_unmodeled  VectorParams1D=off
  Perturbation Torque : Outport
  Perturbation Noise : Outport  Port=2
  wires:
  Add/1 -> Perturbation Torque/1
  Constant/1 -> Add/1
  Constant1/1 -> Add/2
  Constant2/1 -> Add/3
  Constant3/1 -> Add/4
  Constant4/1 -> Add/5
  Constant5/1 -> Add/6

== system attempt_2_Full_Microthruster_Simulation/State Transition Function1/Control Law ==
  note: PLACEHOLDER:
      |
      | Likely only control device on board will be impermanent magnetorquer; TBM if necessary, otherwise leave as zero vector
  In1 : Inport
  Out1 : Outport
  wires:
  In1/1 -> Out1/1

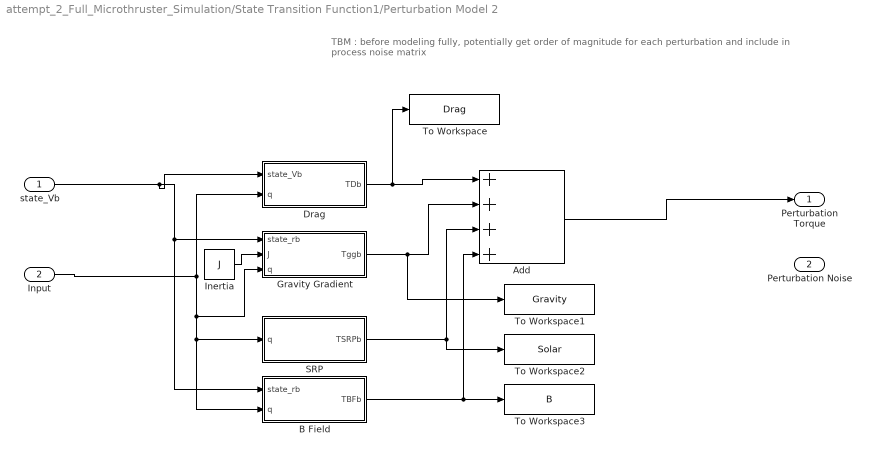
== system attempt_2_Full_Microthruster_Simulation/State Transition Function1/Perturbation Model 2 ==
  note: TBM : before modeling fully, potentially get order of magnitude for each perturbation and include in process noise matrix
  state_Vb : Inport
  Input : Inport  Port=2
  Add : Sum  Inputs=++++
  B Field : Subsystem
  Drag : Subsystem
  Gravity Gradient : Subsystem
  Inertia : Constant  Value=J
  SRP : Subsystem
  To Workspace : ToWorkspace  VariableName=Drag  SaveFormat=Timeseries  SampleTime=-1
  To Workspace1 : ToWorkspace  VariableName=Gravity  SaveFormat=Timeseries  SampleTime=-1
  To Workspace2 : ToWorkspace  VariableName=Solar  SaveFormat=Timeseries  SampleTime=-1
  To Workspace3 : ToWorkspace  VariableName=B  SaveFormat=Timeseries  SampleTime=-1
  Perturbation Torque : Outport
  Perturbation Noise : Outport  Port=2
  wires:
  B Field/1(TBFb) -> To Workspace3/1, Add/4
  Drag/1(TDb) -> To Workspace/1, Add/1
  Input/1 -> B Field/2(q), SRP/1(q), Gravity Gradient/3(q), Drag/2(q)
  Inertia/1 -> Gravity Gradient/2(J)
  Gravity Gradient/1(Tggb) -> To Workspace1/1, Add/2
  state_Vb/1 -> B Field/1(state_rb), Gravity Gradient/1(state_rb), Drag/1(state_Vb)
  SRP/1(TSRPb) -> To Workspace2/1, Add/3
  Add/1 -> Perturbation Torque/1

== system attempt_2_Full_Microthruster_Simulation/State Transition Function1/Unmodeled Perturbations ==
  Add : Sum  Inputs=++++++
  Constant : Constant  Value=drag_unmodeled  VectorParams1D=off
  Constant1 : Constant  Value=grav_grad_unmodeled  VectorParams1D=off
  Constant2 : Constant  Value=mag_field_unmodeled  VectorParams1D=off
  Constant3 : Constant  Value=srp_unmodeled  VectorParams1D=off
  Constant4 : Constant  Value=gr_eff_unmodeled  VectorParams1D=off
  Constant5 : Constant  Value=onboard_unmodeled  VectorParams1D=off
  Perturbation Torque : Outport
  Perturbation Noise : Outport  Port=2
  wires:
  Add/1 -> Perturbation Torque/1
  Constant/1 -> Add/1
  Constant1/1 -> Add/2
  Constant2/1 -> Add/3
  Constant3/1 -> Add/4
  Constant4/1 -> Add/5
  Constant5/1 -> Add/6

== system attempt_2_Full_Microthruster_Simulation/Gyro Sensor Measurement Function/Subsystem/Subsystem ==
  p q r : Inport
  Constant : Constant  Value=dtype_g
  No Dynamics : aerolibnav/Three-axis Gyroscope/Dynamics/No Dynamics  SystemSampleTime=-1  VariantActivationTime=update diagram  Latency=0  AutoFrameSizeCalculation=off
      settings: SourceProductBaseCode=AE
  Subsystem : Subsystem
  Switch : Switch  Threshold=0.5
  "p q r " : Outport  VectorParamsAs1DForOutWhenUnconnected=off
  wires:
  p q r/1 -> Subsystem/1(p q r), No Dynamics/1
  No Dynamics/1 -> Switch/3
  Subsystem/1(Out) -> Switch/1
  Switch/1 -> "p q r "/1
  Constant/1 -> Switch/2

== system attempt_2_Full_Microthruster_Simulation/Gyro Sensor Measurement Function1/Subsystem/Subsystem ==
  p q r : Inport
  Constant : Constant  Value=dtype_g
  No Dynamics : aerolibnav/Three-axis Gyroscope/Dynamics/No Dynamics  SystemSampleTime=-1  VariantActivationTime=update diagram  Latency=0  AutoFrameSizeCalculation=off
      settings: SourceProductBaseCode=AE
  Subsystem : Subsystem
  Switch : Switch  Threshold=0.5
  "p q r " : Outport  VectorParamsAs1DForOutWhenUnconnected=off
  wires:
  p q r/1 -> Subsystem/1(p q r), No Dynamics/1
  No Dynamics/1 -> Switch/3
  Subsystem/1(Out) -> Switch/1
  Switch/1 -> "p q r "/1
  Constant/1 -> Switch/2

== system attempt_2_Full_Microthruster_Simulation/State Transition Function/Perturbation Model 2/B Field ==
  state_rb : Inport
  q : Inport  Port=2
  Clock : Clock
  MATLAB Function : MATLAB Function  TreatAsAtomicUnit=on
  Tb : Scope
  TBFb : Outport
  wires:
  state_rb/1 -> MATLAB Function/1(state_rb)
  q/1 -> MATLAB Function/2(attState)
  MATLAB Function/1(Tmb) -> Tb/1, TBFb/1
  Clock/1 -> MATLAB Function/3(t)

== system attempt_2_Full_Microthruster_Simulation/State Transition Function/Perturbation Model 2/Drag ==
  state_Vb : Inport
  q : Inport  Port=2
  Constant : Constant  Value=geom
  MATLAB Function : MATLAB Function  TreatAsAtomicUnit=on
  Tdrag : Scope
  TDb : Outport
  wires:
  state_Vb/1 -> MATLAB Function/1(state)
  q/1 -> MATLAB Function/2(attState)
  MATLAB Function/1(Td) -> Tdrag/1, TDb/1
  Constant/1 -> MATLAB Function/3(geom)

== system attempt_2_Full_Microthruster_Simulation/State Transition Function/Perturbation Model 2/Gravity Gradient ==
  state_rb : Inport
  J : Inport  Port=2
  q : Inport  Port=3
  MATLAB Function : MATLAB Function  TreatAsAtomicUnit=on
  Tgg : Scope
  Tggb : Outport
  wires:
  state_rb/1 -> MATLAB Function/2(state_rb)
  J/1 -> MATLAB Function/1(J)
  MATLAB Function/1(Tgg) -> Tgg/1, Tggb/1
  q/1 -> MATLAB Function/3(attState)

== system attempt_2_Full_Microthruster_Simulation/State Transition Function/Perturbation Model 2/SRP ==
  q : Inport
  Constant : Constant  Value=geom
  MATLAB Function : MATLAB Function  TreatAsAtomicUnit=on
  Tsrp : Scope
  TSRPb : Outport
  wires:
  MATLAB Function/1(Tsrp) -> Tsrp/1, TSRPb/1
  q/1 -> MATLAB Function/1(attState)
  Constant/1 -> MATLAB Function/2(geom)

== system attempt_2_Full_Microthruster_Simulation/State Transition Function1/Perturbation Model 2/B Field ==
  state_rb : Inport
  q : Inport  Port=2
  Clock : Clock
  MATLAB Function : MATLAB Function  TreatAsAtomicUnit=on
  Tb : Scope
  TBFb : Outport
  wires:
  state_rb/1 -> MATLAB Function/1(state_rb)
  q/1 -> MATLAB Function/2(attState)
  MATLAB Function/1(Tmb) -> Tb/1, TBFb/1
  Clock/1 -> MATLAB Function/3(t)

== system attempt_2_Full_Microthruster_Simulation/State Transition Function1/Perturbation Model 2/Drag ==
  state_Vb : Inport
  q : Inport  Port=2
  Constant : Constant  Value=geom
  MATLAB Function : MATLAB Function  TreatAsAtomicUnit=on
  Tdrag : Scope
  TDb : Outport
  wires:
  state_Vb/1 -> MATLAB Function/1(state)
  q/1 -> MATLAB Function/2(attState)
  MATLAB Function/1(Td) -> Tdrag/1, TDb/1
  Constant/1 -> MATLAB Function/3(geom)

== system attempt_2_Full_Microthruster_Simulation/State Transition Function1/Perturbation Model 2/Gravity Gradient ==
  state_rb : Inport
  J : Inport  Port=2
  q : Inport  Port=3
  MATLAB Function : MATLAB Function  TreatAsAtomicUnit=on
  Tgg : Scope
  Tggb : Outport
  wires:
  state_rb/1 -> MATLAB Function/2(state_rb)
  J/1 -> MATLAB Function/1(J)
  MATLAB Function/1(Tgg) -> Tgg/1, Tggb/1
  q/1 -> MATLAB Function/3(attState)

== system attempt_2_Full_Microthruster_Simulation/State Transition Function1/Perturbation Model 2/SRP ==
  q : Inport
  Constant : Constant  Value=geom
  MATLAB Function : MATLAB Function  TreatAsAtomicUnit=on
  Tsrp : Scope
  TSRPb : Outport
  wires:
  MATLAB Function/1(Tsrp) -> Tsrp/1, TSRPb/1
  q/1 -> MATLAB Function/1(attState)
  Constant/1 -> MATLAB Function/2(geom)

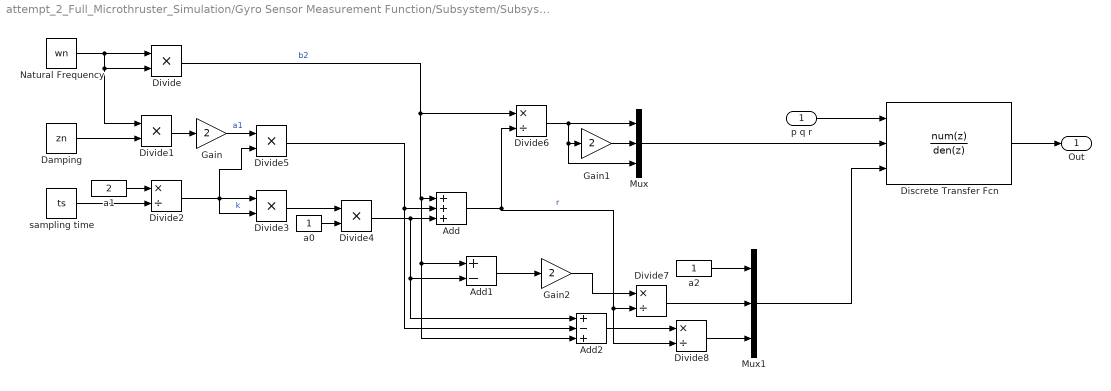
== system attempt_2_Full_Microthruster_Simulation/Gyro Sensor Measurement Function/Subsystem/Subsystem/Subsystem ==
  p q r : Inport
  Add : Sum  Inputs=+++
  Add1 : Sum  Inputs=+-
  Add2 : Sum  Inputs=+-+
  Damping : Constant  Value=zn
  Discrete Transfer Fcn : DiscreteTransferFcn  NumeratorSource=Input port  DenominatorSource=Input port  a0EqualsOne=on
      settings: InputPortMap=u0,p1,p3
  Divide{,1,3..5} (5 alike) : Product  Inputs=**
  Divide{2,6..8} (4 alike) : Product  Inputs=*/
  Gain : Gain  Gain=2
  Gain1 : Gain  Gain=2
  Gain2 : Gain  Gain=2
  Mux : Mux  Inputs=3
  Mux1 : Mux  Inputs=3
  Natural Frequency : Constant  Value=wn
  a0 : Constant
  a1 : Constant  Value=2
  a2 : Constant
  sampling time : Constant  Value=ts
  Out : Outport  VectorParamsAs1DForOutWhenUnconnected=off
  wires:
  a1/1 -> Divide2/1
  Natural Frequency/1 -> Divide/1, Divide/2, Divide1/1
  Divide3/1 -> Divide4/1
  p q r/1 -> Discrete Transfer Fcn/1
  Add1/1 -> Gain2/1
  Gain/1 -> Divide5/1  "a1"
  Damping/1 -> Divide1/2
  a2/1 -> Mux1/1
  Add/1 -> Divide8/2, Divide7/2, Divide6/2  "r"
  a0/1 -> Divide4/2
  Gain2/1 -> Divide7/1
  Mux1/1 -> Discrete Transfer Fcn/3
  Add2/1 -> Divide8/1
  Divide/1 -> Divide6/1, Add2/3, Add1/1, Add/1  "b2"
  Divide8/1 -> Mux1/3
  Divide4/1 -> Add2/1, Add1/2, Add/3
  Divide2/1 -> Divide5/2, Divide3/2, Divide3/1  "k"
  sampling time/1 -> Divide2/2
  Divide1/1 -> Gain/1
  Discrete Transfer Fcn/1 -> Out/1
  Divide5/1 -> Add2/2, Add/2
  Divide7/1 -> Mux1/2
  Mux/1 -> Discrete Transfer Fcn/2
  Divide6/1 -> Mux/3, Gain1/1, Mux/1
  Gain1/1 -> Mux/2

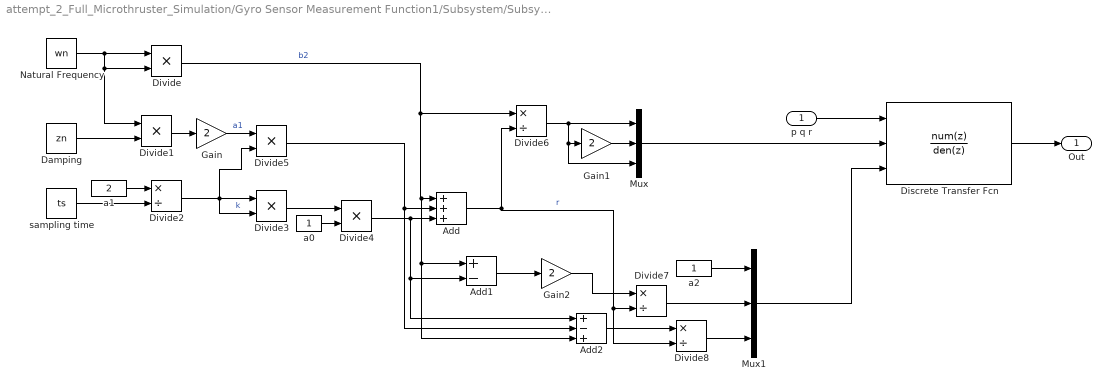
== system attempt_2_Full_Microthruster_Simulation/Gyro Sensor Measurement Function1/Subsystem/Subsystem/Subsystem ==
  p q r : Inport
  Add : Sum  Inputs=+++
  Add1 : Sum  Inputs=+-
  Add2 : Sum  Inputs=+-+
  Damping : Constant  Value=zn
  Discrete Transfer Fcn : DiscreteTransferFcn  NumeratorSource=Input port  DenominatorSource=Input port  a0EqualsOne=on
      settings: InputPortMap=u0,p1,p3
  Divide{,1,3..5} (5 alike) : Product  Inputs=**
  Divide{2,6..8} (4 alike) : Product  Inputs=*/
  Gain : Gain  Gain=2
  Gain1 : Gain  Gain=2
  Gain2 : Gain  Gain=2
  Mux : Mux  Inputs=3
  Mux1 : Mux  Inputs=3
  Natural Frequency : Constant  Value=wn
  a0 : Constant
  a1 : Constant  Value=2
  a2 : Constant
  sampling time : Constant  Value=ts
  Out : Outport  VectorParamsAs1DForOutWhenUnconnected=off
  wires:
  a1/1 -> Divide2/1
  Natural Frequency/1 -> Divide/1, Divide/2, Divide1/1
  Divide3/1 -> Divide4/1
  p q r/1 -> Discrete Transfer Fcn/1
  Add1/1 -> Gain2/1
  Gain/1 -> Divide5/1  "a1"
  Damping/1 -> Divide1/2
  a2/1 -> Mux1/1
  Add/1 -> Divide8/2, Divide7/2, Divide6/2  "r"
  a0/1 -> Divide4/2
  Gain2/1 -> Divide7/1
  Mux1/1 -> Discrete Transfer Fcn/3
  Add2/1 -> Divide8/1
  Divide/1 -> Divide6/1, Add2/3, Add1/1, Add/1  "b2"
  Divide8/1 -> Mux1/3
  Divide4/1 -> Add2/1, Add1/2, Add/3
  Divide2/1 -> Divide5/2, Divide3/2, Divide3/1  "k"
  sampling time/1 -> Divide2/2
  Divide1/1 -> Gain/1
  Discrete Transfer Fcn/1 -> Out/1
  Divide5/1 -> Add2/2, Add/2
  Divide7/1 -> Mux1/2
  Mux/1 -> Discrete Transfer Fcn/2
  Divide6/1 -> Mux/3, Gain1/1, Mux/1
  Gain1/1 -> Mux/2

== matlab function attempt_2_Full_Microthruster_Simulation/Sun Sensor ==
  data: xk input; y output; JD_start input; sim_time input; sigma_s input; sigma_q input; y_no_noise output
function [y,y_no_noise] = sunVec(xk,JD_start,sim_time,sigma_s,sigma_q)

JD_new = JD_start + sim_time/3600/24; % add sim time in days to start time

q = xk(4:7);
eps = q(1:3);
eta = q(4);

jul_cent = (JD_new-2451545)/36525; % julian centuries since 2000
lambda_S = wrapTo360(280.4606184 + 36000.77005361*jul_cent); % mean longitude of sun in deg
M_S = wrapTo360(357.5277233 + 35999.05034*jul_cent); % mean anomaly of sun in deg
lambda_e = wrapTo180(lambda_S + 1.914666471*sind(M_S) + 0.019994643*sind(2*M_S)); % ecliptic long of sun in deg

eps_sun = 23.439291-0.0130042*jul_cent;
sun_ECI = [cosd(lambda_e); cosd(eps_sun)*sind(lambda_e); sind(eps_sun)*sind(lambda_e)];


% Calculate Y(a,q) for sun sensor
Y_s = [eta*eye(3)-Functions.vec2cross(eps) -eps]*[Functions.vec2cross(sun_ECI) sun_ECI;
                                                      -sun_ECI'                    0];

coder.extrinsic('randn');
v_k = zeros([3 1]); %#ok<*PREALL> simulink needs this to determine variable size
v_k = randn(3,1)*sigma_q;   
m_k = zeros([3 1]);
m_k = [randn(3,1)*sigma_s];
y_no_noise = [zeros(3) Y_s]*xk; 
y = y_no_noise + m_k; % measurement with measurement noise
